simulink model "DVNonlineairelinmod"  (Simulink 8.5)
settings: Solver=ode45  StartTime=0.0  StopTime=6  RelTol=1e-3
values from neighbouring files (symbols this model uses):
  br = 0.001    [Correcteur.mat]    (also in DVinitialisation.m; QFT.m)
  Cm0 = 42.8155296593    [Correcteur.mat]    (also in DVinitialisation.m = r0*FXE+br*W0; QFT.m = r0*FXE+br*W0)
  Cx = 0.5    [Correcteur.mat]    (also in DVinitialisation.m; QFT.m)
  Fz = 1962    [Correcteur.mat]    (also in DVinitialisation.m; QFT.m = m*g; pacejka_BE_Matlab_fnc.m = in(3))
  g = 9.81    [Correcteur.mat]    (also in DVinitialisation.m; QFT.m)
  J = 1    [Correcteur.mat]    (also in DVinitialisation.m; QFT.m)
  K = 125    [Correcteur.mat]    (also in DVinitialisation.m; PIDF_Design.m = K/M; QFT.m)
  lambda0 = 0.0136    [Correcteur.mat]    (also in DVinitialisation.m; QFT.m)
  lambda2 = 4e-08    [Correcteur.mat]    (also in DVinitialisation.m; QFT.m)
  m = 200    [Correcteur.mat]    (also in DVinitialisation.m; QFT.m = var1(i1))
  mu = 1    [Correcteur.mat]    (also in DVinitialisation.m; QFT.m = var2(i2); pacejka_BE_Matlab_fnc.m = in(4))
  pneu = [1.712 -66.87 1169 851.9 4.943 0.01399 -0.1911 1 0.972 0 0.186 0.22 ... (35 elements, 1x35)]    [Correcteur.mat]    (also in DVinitialisation.m = [a0,a1,a2,a3,a4,a5,a6,a7,am0,am1,am2,am3,am4,am5,am6,am7,am8; pacejka_BE_Matlab_fnc.m = in(5:end); param_pneu_P1_OK.m = [a0,a1,a2,a3,a4,a5,a6,a7,am0,am1,am2,am3,am4,am5,am6,am7,am8)
  r0 = 0.3    [Correcteur.mat]    (also in DVinitialisation.m; QFT.m)
  ro = 1.225    [Correcteur.mat]    (also in DVinitialisation.m; QFT.m)
  Sx = 1    [Correcteur.mat]    (also in DVinitialisation.m; QFT.m)
  VMAX = 55.5555555556    [Correcteur.mat]    (also in DVinitialisation.m; QFT.m)
  VMIN = 0.138888888889    [Correcteur.mat]    (also in DVinitialisation.m; QFT.m)
  Vx0 = 19.4444444444    [Correcteur.mat]    (also in DVinitialisation.m; QFT.m = var3(i3))
  W0 = 64.9781778438    [Correcteur.mat]    (also in DVinitialisation.m = 1/r0*(Vx0/(1-(Te/100))); QFT.m = 1/r0*(Vx0/(1-(Te/100))))
  WMAX = 185.185185185    [Correcteur.mat]    (also in DVinitialisation.m; QFT.m)
  WMIN = 0    [Correcteur.mat]    (also in DVinitialisation.m; QFT.m)
settings Model: Creator=StephaneBarroso  LastModifiedBy=StephaneBarroso
settings DataIOCC: SignalLoggingSaveFormat=Dataset
settings OptimizationCC: ExpressionDepthLimit=128
settings DebuggingCC: UnderspecifiedInitializationDetection=Simplified  MergeDetectMultiDrivingBlocksExec=error  FcnCallInpInsideContextMsg=EnableAllAsError  StateNameClashWarn=none
settings GRTTargetCC: CombineOutputUpdateFcns=on  GRTInterface=off

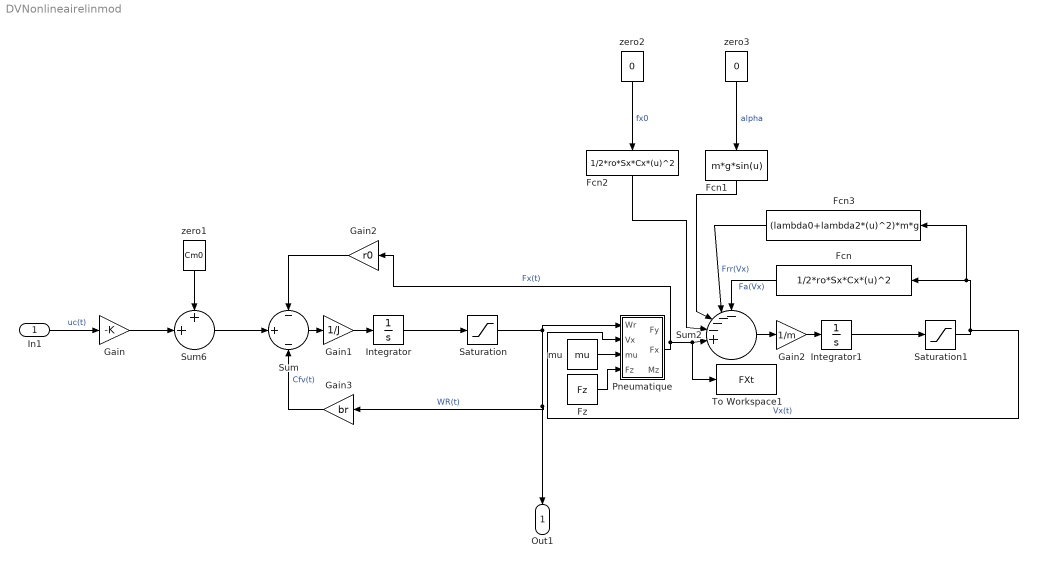
== system DVNonlineairelinmod ==
  In1 : Inport
  Fcn : Fcn  Expr=1/2*ro*Sx*Cx*(u)^2
  Fcn1 : Fcn  Expr=m*g*sin(u)
  Fcn2 : Fcn  Expr=1/2*ro*Sx*Cx*(u)^2
  Fcn3 : Fcn  Expr=(lambda0+lambda2*(u)^2)*m*g
  Fz : Constant  Value=Fz
  Gain : Gain  Gain=-K
  Gain1 : Gain  Gain=1/J
  Gain2 : Gain  Gain=r0
  "Gain2 " : Gain  Gain=1/m
  Gain3 : Gain  Gain=br
  Integrator : Integrator  InitialCondition=W0
  Integrator1 : Integrator  InitialCondition=Vx0
  Pneumatique : Subsystem
  Saturation : Saturate  UpperLimit=WMAX  LowerLimit=WMIN
  Saturation1 : Saturate  UpperLimit=VMAX  LowerLimit=VMIN
  Sum : Sum  Inputs=-|+|-
  Sum2 : Sum  Inputs=----+|||
  Sum6 : Sum  Inputs=++|
  To Workspace1 : ToWorkspace  VariableName=FXt  SaveFormat=Timeseries  SampleTime=-1
  mu : Constant  Value=mu
  zero1 : Constant  Value=Cm0
  zero2 : Constant  Value=0
  zero3 : Constant  Value=0
  Out1 : Outport
  wires:
  zero1/1 -> Sum6/1
  Gain/1 -> Sum6/2
  In1/1 -> Gain/1  "uc(t)"
  Fz/1 -> Pneumatique/4("Fz ")
  mu/1 -> Pneumatique/3("mu ")
  Gain2/1 -> Sum/1
  Saturation/1 -> Gain3/1, Out1/1, Pneumatique/1(Wr)  "WR(t)"
  Integrator/1 -> Saturation/1
  Gain1/1 -> Integrator/1
  Saturation1/1 -> Pneumatique/2(Vx), Fcn3/1, Fcn/1  "Vx(t)"
  Fcn1/1 -> Sum2/3
  "Gain2 "/1 -> Integrator1/1
  Gain3/1 -> Sum/3  "Cfv(t)"
  Integrator1/1 -> Saturation1/1
  Fcn2/1 -> Sum2/4
  Fcn3/1 -> Sum2/2  "Frr(Vx)"
  Sum2/1 -> "Gain2 "/1
  Fcn/1 -> Sum2/1  "Fa(Vx)"
  Sum/1 -> Gain1/1
  Sum6/1 -> Sum/2
  Pneumatique/2(Fx) -> Gain2/1, To Workspace1/1, Sum2/5  "Fx(t)"
  zero2/1 -> Fcn2/1  "fx0"
  zero3/1 -> Fcn1/1  "alpha"

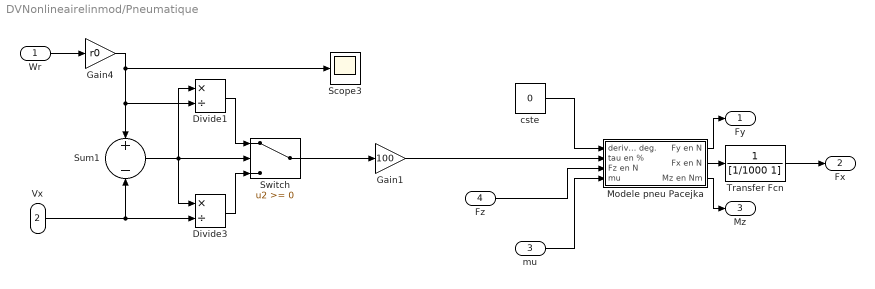
== system DVNonlineairelinmod/Pneumatique ==
  Wr : Inport
  Vx : Inport  Port=2
  "mu " : Inport  Port=3
  "Fz " : Inport  Port=4
  Divide1 : Product  Inputs=*/
  Divide3 : Product  Inputs=*/
  Gain1 : Gain  Gain=100
  Gain4 : Gain  Gain=r0
  Modele pneu Pacejka : Subsystem
  Scope3 : Scope
  Sum1 : Sum  Inputs=+-
  Switch : Switch
  Transfer Fcn : TransferFcn  Denominator=[1/1000 1]
  cste : Constant  Value=0
  Fy : Outport
  Fx : Outport  Port=2
  Mz : Outport  Port=3
  wires:
  "Fz "/1 -> Modele pneu Pacejka/3(Fz en N)
  "mu "/1 -> Modele pneu Pacejka/4(mu)
  Gain4/1 -> Scope3/1, Divide1/2, Sum1/1
  Modele pneu Pacejka/3(Mz en Nm) -> Mz/1
  Modele pneu Pacejka/1(Fy en N) -> Fy/1
  Vx/1 -> Divide3/2, Sum1/2
  Modele pneu Pacejka/2(Fx en N) -> Transfer Fcn/1
  Wr/1 -> Gain4/1
  cste/1 -> Modele pneu Pacejka/1(deriv. en deg.)
  Sum1/1 -> Divide3/1, Divide1/1, Switch/2
  Divide1/1 -> Switch/1
  Divide3/1 -> Switch/3
  Gain1/1 -> Modele pneu Pacejka/2(tau en %)
  Switch/1 -> Gain1/1
  Transfer Fcn/1 -> Fx/1

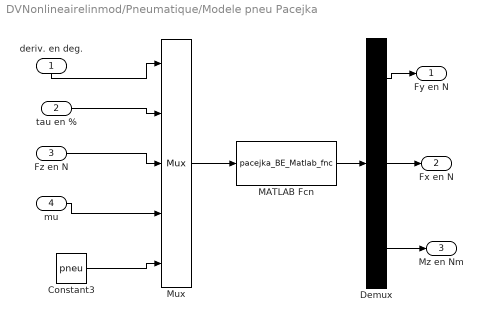
== system DVNonlineairelinmod/Pneumatique/Modele pneu Pacejka ==
  deriv. en deg. : Inport
  tau en % : Inport  Port=2
  Fz en N : Inport  Port=3
  mu : Inport  Port=4
  Constant3 : Constant  Value=pneu
  Demux : Demux  Outputs=3
  MATLAB Fcn : MATLABFcn  MATLABFcn=pacejka_BE_Matlab_fnc  OutputDimensions=3
  Mux : Mux  Inputs=5
  Fy en N : Outport
  Fx en N : Outport  Port=2
  Mz en Nm : Outport  Port=3
  wires:
  MATLAB Fcn/1 -> Demux/1
  Mux/1 -> MATLAB Fcn/1
  deriv. en deg./1 -> Mux/1
  Demux/1 -> Fy en N/1
  Demux/2 -> Fx en N/1
  Demux/3 -> Mz en Nm/1
  tau en %/1 -> Mux/2
  Fz en N/1 -> Mux/3
  mu/1 -> Mux/4
  Constant3/1 -> Mux/5
